simulink model "simlink13"  (R2017b)
settings: Solver=VariableStepAuto  StartTime=0.0  StopTime=10  RelTol=1e-3
PreLoadFcn:
  | init.m;
values from neighbouring files (symbols this model uses):
  gama1 = ones(1001,1)*55    [init.m]    (also in int.m = 100; workspace.m = ones(1001,1)*200)
  gama2 = ones(1001,1)*10    [init.m]    (also in int.m = 200; sample_sim.m = gama2+ones(1001,1)*5; workspace.m = ones(1001,1)*5)
settings Model: Creator=Administrator  LastModifiedBy=Administrator
settings SolverCC: ZeroCrossAlgorithm=Adaptive
settings DebuggingCC: MaxConsecutiveZCsMsg=none

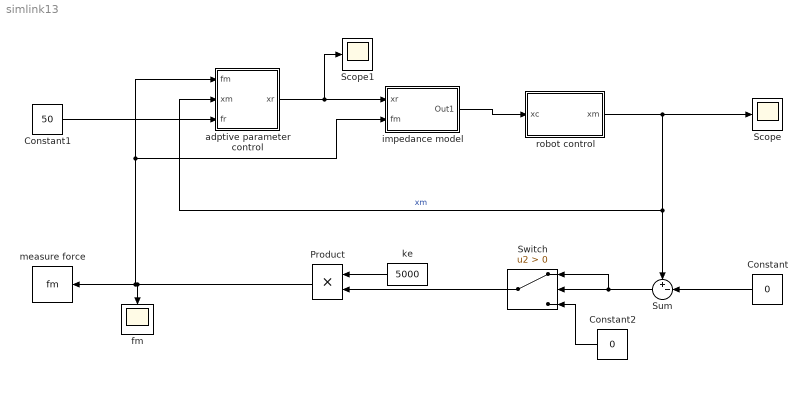
== system simlink13 ==
  Constant : Constant  Value=0
  Constant1 : Constant  Value=50
  Constant2 : Constant  Value=0
  Product : Product
  Scope : Scope
  Scope1 : Scope
  Sum : Sum  Inputs=+-|
  Switch : Switch  Criteria=u2 > Threshold
  adptive parameter control : Subsystem
  fm : Scope
  impedance model : Subsystem
  ke : Constant  Value=5000
  "measure force " : ToWorkspace  VariableName=fm  SaveFormat=Timeseries  SampleTime=-1
  robot control : Subsystem
  wires:
  Constant1/1 -> adptive parameter control/3(fr)
  Product/1 -> "measure force "/1, impedance model/2(fm), adptive parameter control/1(fm), fm/1
  robot control/1("xm ") -> adptive parameter control/2(xm), Sum/1, Scope/1  "xm"
  impedance model/1(Out1) -> robot control/1(xc)
  ke/1 -> Product/1
  adptive parameter control/1(xr) -> Scope1/1, impedance model/1(xr)
  Constant/1 -> Sum/2
  Sum/1 -> Switch/1, Switch/2
  Switch/1 -> Product/2
  Constant2/1 -> Switch/3

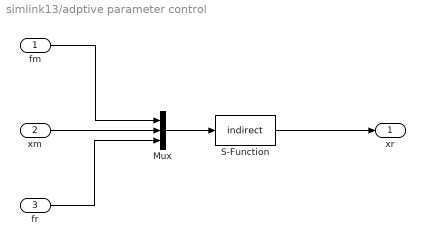
== system simlink13/adptive parameter control ==
  fm : Inport
  xm : Inport  Port=2
  fr : Inport  Port=3
  Mux : Mux  Inputs=3
  S-Function : S-Function  FunctionName=indirect  Parameters=gama1 gama2 kd  SFunctionDeploymentMode=off  EnableBusSupport=off
  xr : Outport
  wires:
  fm/1 -> Mux/1
  xm/1 -> Mux/2
  Mux/1 -> S-Function/1
  S-Function/1 -> xr/1
  fr/1 -> Mux/3

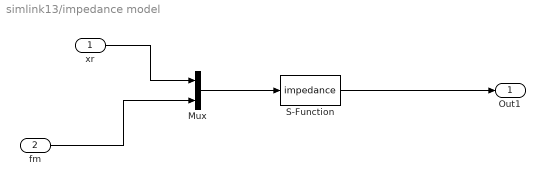
== system simlink13/impedance model ==
  xr : Inport
  fm : Inport  Port=2
  Mux : Mux  Inputs=2
  S-Function : S-Function  FunctionName=impedance  Parameters=bd kd  SFunctionDeploymentMode=off  EnableBusSupport=off
  Out1 : Outport
  wires:
  xr/1 -> Mux/1
  Mux/1 -> S-Function/1
  S-Function/1 -> Out1/1
  fm/1 -> Mux/2

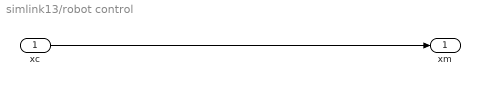
== system simlink13/robot control ==
  xc : Inport
  "xm " : Outport
  wires:
  xc/1 -> "xm "/1
